simulink model "system_integration"  (R2021a)
settings: Solver=VariableStepAuto  StartTime=0.0  StopTime=3600*5  RelTol=1e-3
undefined symbols (not defined in the file): Ion, Lithium
libraries: spsSeriesRLCBranchLib x10, spsMosfetLib x7, spsBatteryLib x6, spsVoltageMeasurementLib x6, spsBreakerLib x3, spsCurrentMeasurementLib x3, spspowerguiLib x2, spsDCMachineLib x1, spsDiodeLib x1, spsPVArrayLib x1
settings Model: Creator=hp  LastModifiedBy=hp

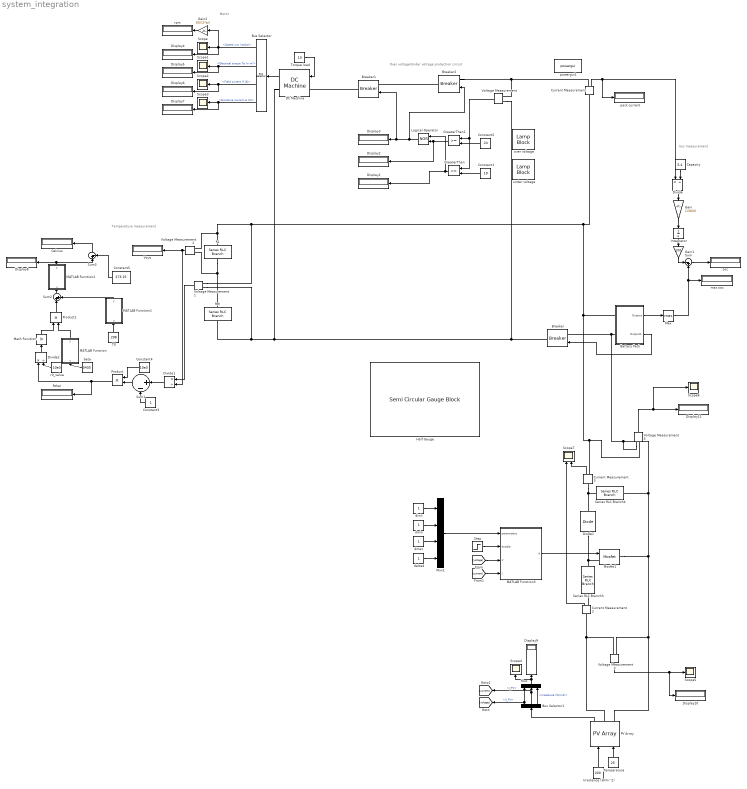
== system system_integration ==
  note: Temperature measurement
  note: Soc measurement
  note: Over voltage/Under voltage protection circuit
  note: Motor
  Battery Pack : Subsystem
  Breaker : spsBreakerLib/Breaker  InitialState=0  SwitchingTimes="[1/60  5/60]"  External=on  BreakerResistance=0.01  SnubberResistance=1e6  SnubberCapacitance=inf  Measurements=None  MoreParameters=on  NoBreakLoop=off
      settings: SourceProductBaseCode=PS
  Breaker1 : spsBreakerLib/Breaker  InitialState=0  SwitchingTimes="[1/60  5/60]"  External=on  BreakerResistance=0.01  SnubberResistance=1e6  SnubberCapacitance=inf  Measurements=None  MoreParameters=on  NoBreakLoop=off
      settings: SourceProductBaseCode=PS
  Breaker2 : spsBreakerLib/Breaker  InitialState=0  SwitchingTimes="[1/60  5/60]"  External=on  BreakerResistance=0.01  SnubberResistance=1e6  SnubberCapacitance=inf  Measurements=None  MoreParameters=on  NoBreakLoop=off
      settings: SourceProductBaseCode=PS
  Bus Selector : BusSelector  OutputSignals=Speed wm (rad/s),Electrical torque Te (n m),Field current if (A),Armature current ia (A)
  Bus Selector1 : BusSelector  OutputSignals=V_PV,I_PV,Irradiance (W/m2)
  Capacity : Constant  Value=5.4
  Celcius : Display
  Constant1 : Constant  Value=19
  Constant2 : Constant  Value=24
  Constant3 : Constant
  Constant4 : Constant  Value=10e3
  Constant5 : Constant  Value=273.15
  Current Measurement : spsCurrentMeasurementLib/Current Measurement  PhasorSimulation=off  OutputType=Complex  PSBequivalent=0
  Current Measurement2 : spsCurrentMeasurementLib/Current Measurement  PhasorSimulation=off  OutputType=Complex  PSBequivalent=0
  Current Measurement3 : spsCurrentMeasurementLib/Current Measurement  PhasorSimulation=off  OutputType=Complex  PSBequivalent=0
  DC Machine : spsDCMachineLib/DC Machine  PresetModel=No  MechanicalLoad=Torque TL  FieldType=Permanent magnet  ShowDetailedParameters=on  MeasurementBus=off  RLa="[ 0.6  0.012]"  RLf="[ 240  120]"  Laf=1.8  MachineConstant=Torque constant (N.m/A)  Ke=1.8  Kt=1.8  J=1  Bm=0  Tf=0  w0=1  Ifinit=1  TsPowergui=0  TsBlock=-1
  Diode1 : spsDiodeLib/Diode  Ron=0.001  Lon=0  Vf=0.8  IC=0  UseSnubber=0  Rs=500  Cs=250e-9  Measurements=off
  Display{1..11} (11 alike) : Display
  Divide : Product  Inputs=*/
  Divide1 : Product  Inputs=*/
  Divide2 : Product  Inputs=*/
  Gain : Gain  Gain=1/3600
  Gain1 : Gain  Gain=100
  Gain2 : Gain  Gain=60/(2*pi)
  GreaterThan : RelationalOperator  Operator=<=  OutDataTypeStr=boolean  RndMeth=Simplest
  GreaterThan1 : RelationalOperator  OutDataTypeStr=boolean  RndMeth=Simplest
  Half Gauge : SemiCircularGaugeBlock
  Integrator : Integrator
  Irradiance (W/m^2) : Constant  Value=200
  Logical Operator : Logic  Operator=NOR  AllPortsSameDT=off  OutDataTypeStr=boolean
  MATLAB Function : MATLAB Function  TreatAsAtomicUnit=on
  MATLAB Function1 : MATLAB Function  TreatAsAtomicUnit=on
  MATLAB Function2 : MATLAB Function  TreatAsAtomicUnit=on
  MATLAB Function3 : MATLAB Function  TreatAsAtomicUnit=on
  Math Function : Math  Operator=log  SaturateOnIntegerOverflow=on
  Max : MinMax  Function=max
  Mosfet1 : spsMosfetLib/Mosfet  Ron=0.1  Lon=0  Rd=0.01  Vfd=0  IC=0  Rs=1e5  Cs=inf  Measurements=off
  Mux : Mux  Inputs=3
  Mux1 : Mux
  PV Array : spsPVArrayLib/PV Array  Npar=40  Nser=10  PlotType=array @ 1000 W/m2 & specified temperatures  S_vec="[ 1000  500  100 ]"  Temp_C_vec=[45 25]  ModuleName=A10Green Technology A10J-S72-180  PlotWhenSelected=off  Pm=179.928  Ncell=72  Voc=44.06  Isc=5.31  Vm=36.72  Im=4.9  beta_Voc_pc=-0.3616  alpha_Isc_pc=0.041507  beta_Voc=-0.15932  alpha_Isc=0.002204  IL=5.3186  I0=1.8308e-10  nI=0.99015  Rsh=227.068  Rs=0.36738  RobustModel=off  RobustCellTemperature=313.3991  BAL=on  Tc=1e-6  Tfilter=5e-5
  Product : Product
  Product1 : Product
  R1 : spsSeriesRLCBranchLib/Series RLC Branch  LConnTagsString=__new0  RConnTagsString=__new0  BranchType=R  Resistance=10e3  Inductance=1e-3  SetiL0=off  InitialCurrent=0  Capacitance=1e-6  Setx0=off  InitialVoltage=0  Measurements=None
  Rth : spsSeriesRLCBranchLib/Series RLC Branch  LConnTagsString=__new0  RConnTagsString=__new0  BranchType=R  Resistance=5625  Inductance=1e-3  SetiL0=off  InitialCurrent=0  Capacitance=1e-6  Setx0=off  InitialVoltage=0  Measurements=None
  Rther : Display
  Scope{,1..6} (7 alike) : Scope
  Scope7 : Scope  NumInputPorts=2
  Series RLC Branch3 : spsSeriesRLCBranchLib/Series RLC Branch  LConnTagsString=__new0  RConnTagsString=__new0  BranchType=L  Resistance=1  Inductance=1e-3  SetiL0=off  InitialCurrent=0  Capacitance=1e-6  Setx0=off  InitialVoltage=0  Measurements=None
  Series RLC Branch4 : spsSeriesRLCBranchLib/Series RLC Branch  LConnTagsString=__new0  RConnTagsString=__new0  BranchType=C  Resistance=1  Inductance=1e-3  SetiL0=off  InitialCurrent=0  Capacitance=100e-6  Setx0=off  InitialVoltage=0  Measurements=None
  Step : Step  Time=0.0001  SampleTime=0
  Sum : Sum  Inputs=|-+
  Sum1 : Sum  Inputs=|+-
  Sum2 : Sum  Inputs=|++
  Sum3 : Sum  Inputs=|+-
  T0 : Constant  Value=298
  Temperature : Constant  Value=25
  Torque load : Constant  Value=10
  Voltage Measurement{,1..4} (5 alike) : spsVoltageMeasurementLib/Voltage Measurement  PhasorSimulation=off  OutputType=Complex  PSBequivalent=0
  Vout : Display
  beta : Constant  Value=3435
  deltad : Constant
  dinit : Constant
  dmax : Constant
  dmin : Constant
  max soc : Display
  over voltage : LampBlock
  pack current : Display
  powergui1 : spspowerguiLib/powergui  Priority=1  SimulationMode=Discrete  SampleTime=100e-6  frequency=60  Iterations=50  frequencyindice=0  Pbase=100e6  ErrMax=1e-4  UnitsV=kV  UnitsW=MW  buscounter=0  FunctionMessages=off  echomessages=off  EnableUseOfTLC=off  CurrentSourceSwitches=off  DisableSnubberDevices=off  DisableRonSwitches=off  DisableVfSwitches=off  DisplayEquations=off  AutomaticDiscreteSolvers=off  SolverType=Tustin/Backward Euler (TBE)  Interpol=off  ExternalGateDelay=off  methode=off  Ts=100  x0status=blocks  SPID=on  SwTol=0  HookPort=off  NonlinearTolerance=1e-4  nMaxIteration=100  ContinueOnMaxIteration=off  RestoreLinks=warning  ResistiveCurrentMeasurement=off  Frange=[0:2:500]  Ylog=off  Xlog=on  ShowGrid=off  save=off  variable=ZData  structure=0  ZoomFFT=off  StartTime=0.0  cycles=1  DisplayStyle=1  fundamental=60  FreqAxis=off  MaxFrequency=1000  frequencyindicesteady=1  RmsSteady=1  display=off
  r0_value : Constant  Value=10e3
  rpm : Display
  soc : Display
  under voltage : LampBlock
  wires:
  Capacity/1 -> Divide/2
  Current Measurement/1 -> pack current/1, Divide/1
  Divide/1 -> Gain/1
  Gain/1 -> Integrator/1
  Max/1 -> Sum/2, max soc/1
  Battery Pack/1(Outport) -> Max/1
  Sum/1 -> soc/1
  Integrator/1 -> Gain1/1
  Gain1/1 -> Sum/1
  Voltage Measurement/1 -> GreaterThan1/1, GreaterThan/1
  Constant1/1 -> GreaterThan/2
  Constant2/1 -> GreaterThan1/2
  GreaterThan/1 -> Display1/1, Logical Operator/1
  GreaterThan1/1 -> Display2/1, Logical Operator/2
  Logical Operator/1 -> Breaker2/1, Breaker1/1, Display3/1
  Bus Selector/4 -> Display7/1, Scope3/1  "<Armature current ia (A)>"
  Bus Selector/3 -> Display6/1, Scope2/1  "<Field current if (A)>"
  DC Machine/1 -> Bus Selector/1
  Bus Selector/2 -> Display5/1, Scope1/1  "<Electrical torque Te (n m)>"
  Gain2/1 -> rpm/1
  Bus Selector/1 -> Gain2/1, Display4/1, Scope/1  "<Speed wm (rad/s)>"
  Divide2/1 -> Math Function/1
  MATLAB Function2/1(y) -> Sum3/1, Display8/1
  Sum3/1 -> Celcius/1
  Constant5/1 -> Sum3/2
  Sum1/1 -> Product/2
  Product/1 -> Rther/1, Divide2/1
  Voltage Measurement1/1 -> Divide1/1
  beta/1 -> MATLAB Function/1(u)
  Constant4/1 -> Product/1
  Voltage Measurement2/1 -> Vout/1, Divide1/2
  T0/1 -> MATLAB Function1/1(u)
  Constant3/1 -> Sum1/2
  MATLAB Function1/1(y) -> Sum2/2
  Sum2/1 -> MATLAB Function2/1(u)
  r0_value/1 -> Divide2/2
  Product1/1 -> Sum2/1
  Divide1/1 -> Sum1/1
  Torque load/1 -> DC Machine/1
  MATLAB Function/1(y) -> Product1/2
  Math Function/1 -> Product1/1
  Battery Pack/2(Outport1) -> Breaker/1
  Mux/1 -> Scope4/1, Display9/1
  [voltage] -> MATLAB Function3/3(V)
  Step/1 -> MATLAB Function3/2(enable)
  Voltage Measurement4/1 -> Scope6/1, Display11/1
  dinit/1 -> Mux1/1
  Bus Selector1/3 -> Mux/3  "<Irradiance (W/m2)>"
  [current] -> MATLAB Function3/4(I)
  Mux1/1 -> MATLAB Function3/1(parameters)
  Bus Selector1/1 -> Mux/1, [voltage]  "<V_PV>"
  Temperature/1 -> PV Array/2
  Voltage Measurement3/1 -> Display10/1, Scope5/1
  Current Measurement2/1 -> Scope7/1
  dmin/1 -> Mux1/2
  Current Measurement3/1 -> Scope7/2
  deltad/1 -> Mux1/4
  dmax/1 -> Mux1/3
  Irradiance (W/m^2)/1 -> PV Array/1
  PV Array/1 -> Bus Selector1/1
  Bus Selector1/2 -> Mux/2, [current]  "<I_PV>"
  MATLAB Function3/1(d) -> Mosfet1/1
  connections:
  Voltage Measurement1/LConn2 -- Breaker/RConn1 -- Voltage Measurement/LConn2 -- DC Machine/RConn1 -- Rth/RConn1
  Breaker2/LConn1 -- Current Measurement/RConn1 -- Voltage Measurement/LConn1
  Breaker1/RConn1 -- DC Machine/LConn1
  Breaker2/RConn1 -- Breaker1/LConn1
  R1/RConn1 -- Rth/LConn1 -- Voltage Measurement2/LConn2
  Current Measurement3/RConn1 -- Current Measurement/LConn1 -- Voltage Measurement1/LConn1 -- Voltage Measurement2/LConn1 -- R1/LConn1 -- Battery Pack/LConn1 -- Voltage Measurement4/LConn1
  Voltage Measurement4/LConn2 -- Mosfet1/RConn1 -- Voltage Measurement3/LConn2 -- PV Array/RConn2 -- Series RLC Branch4/RConn1 -- Battery Pack/LConn2 -- Breaker/LConn1
  Voltage Measurement3/LConn1 -- PV Array/RConn1 -- Current Measurement2/LConn1
  Mosfet1/LConn1 -- Diode1/LConn1 -- Series RLC Branch3/RConn1
  Current Measurement3/LConn1 -- Series RLC Branch4/LConn1 -- Diode1/RConn1
  Current Measurement2/RConn1 -- Series RLC Branch3/LConn1

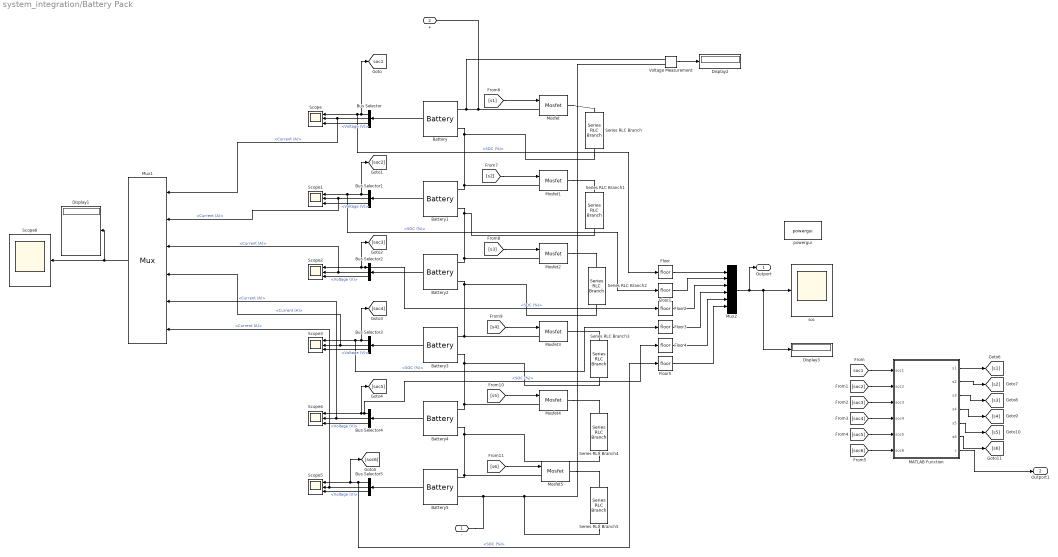
== system system_integration/Battery Pack ==
  Battery : spsBatteryLib/Battery  BatType=Lithium-Ion  ShowTempParam=off  ThermalPreset=no  ShowAgeParam=off  NomV=3.7  NomQ=5.4  SOC=65  Batt_Tr=30  PresetModel=on  MaxQ=5.4  MinV=2.775  FullV=4.3068  Dis_rate=2.3478  R=0.0068519  Normal_OP=4.8835  expZone="[3.9974      0.2653]"  current=[6.5 13 32.5]  Units=Time  Tci=20  NomT=20  T2=-30  MaxQ2=4.8  FullV2=7.1  Normal_OP2=5.655  expZone2="[6.58           1]"  Rca=0.6  ti=2000  Dp=0  Neq0=0  Tsim=1e6  Ta1=25  Qeol=5.4*0.9  Reol=0.013333*1.2  Char_age=[2.3478, 3]  Dis_age=[2.3478, 10]  N1=1500  N2=10500  N3=1000  N4=1400  Ta2=45  N5=950
  Battery1 : spsBatteryLib/Battery  BatType=Lithium-Ion  ShowTempParam=off  ThermalPreset=no  ShowAgeParam=off  NomV=3.7  NomQ=5.4  SOC=63  Batt_Tr=30  PresetModel=on  MaxQ=5.4  MinV=2.775  FullV=4.3068  Dis_rate=2.3478  R=0.0068519  Normal_OP=4.8835  expZone="[3.9974      0.2653]"  current=[6.5 13 32.5]  Units=Time  Tci=20  NomT=20  T2=-30  MaxQ2=4.8  FullV2=7.1  Normal_OP2=5.655  expZone2="[6.58           1]"  Rca=0.6  ti=2000  Dp=0  Neq0=0  Tsim=1e6  Ta1=25  Qeol=5.4*0.9  Reol=0.013333*1.2  Char_age=[2.3478, 3]  Dis_age=[2.3478, 10]  N1=1500  N2=10500  N3=1000  N4=1400  Ta2=45  N5=950
  Battery2 : spsBatteryLib/Battery  BatType=Lithium-Ion  ShowTempParam=off  ThermalPreset=no  ShowAgeParam=off  NomV=3.7  NomQ=5.4  SOC=64  Batt_Tr=30  PresetModel=on  MaxQ=5.4  MinV=2.775  FullV=4.3068  Dis_rate=2.3478  R=0.0068519  Normal_OP=4.8835  expZone="[3.9974      0.2653]"  current=[6.5 13 32.5]  Units=Time  Tci=20  NomT=20  T2=-30  MaxQ2=4.8  FullV2=7.1  Normal_OP2=5.655  expZone2="[6.58           1]"  Rca=0.6  ti=2000  Dp=0  Neq0=0  Tsim=1e6  Ta1=25  Qeol=5.4*0.9  Reol=0.013333*1.2  Char_age=[2.3478, 3]  Dis_age=[2.3478, 10]  N1=1500  N2=10500  N3=1000  N4=1400  Ta2=45  N5=950
  Battery3 : spsBatteryLib/Battery  BatType=Lithium-Ion  ShowTempParam=off  ThermalPreset=no  ShowAgeParam=off  NomV=3.7  NomQ=5.4  SOC=62  Batt_Tr=30  PresetModel=on  MaxQ=5.4  MinV=2.775  FullV=4.3068  Dis_rate=2.3478  R=0.0068519  Normal_OP=4.8835  expZone="[3.9974      0.2653]"  current=[6.5 13 32.5]  Units=Time  Tci=20  NomT=20  T2=-30  MaxQ2=4.8  FullV2=7.1  Normal_OP2=5.655  expZone2="[6.58           1]"  Rca=0.6  ti=2000  Dp=0  Neq0=0  Tsim=1e6  Ta1=25  Qeol=5.4*0.9  Reol=0.013333*1.2  Char_age=[2.3478, 3]  Dis_age=[2.3478, 10]  N1=1500  N2=10500  N3=1000  N4=1400  Ta2=45  N5=950
  Battery4 : spsBatteryLib/Battery  BatType=Lithium-Ion  ShowTempParam=off  ThermalPreset=no  ShowAgeParam=off  NomV=3.7  NomQ=5.4  SOC=66  Batt_Tr=30  PresetModel=on  MaxQ=5.4  MinV=2.775  FullV=4.3068  Dis_rate=2.3478  R=0.0068519  Normal_OP=4.8835  expZone="[3.9974      0.2653]"  current=[6.5 13 32.5]  Units=Time  Tci=20  NomT=20  T2=-30  MaxQ2=4.8  FullV2=7.1  Normal_OP2=5.655  expZone2="[6.58           1]"  Rca=0.6  ti=2000  Dp=0  Neq0=0  Tsim=1e6  Ta1=25  Qeol=5.4*0.9  Reol=0.013333*1.2  Char_age=[2.3478, 3]  Dis_age=[2.3478, 10]  N1=1500  N2=10500  N3=1000  N4=1400  Ta2=45  N5=950
  Battery5 : spsBatteryLib/Battery  BatType=Lithium-Ion  ShowTempParam=off  ThermalPreset=no  ShowAgeParam=off  NomV=3.7  NomQ=5.4  SOC=65  Batt_Tr=30  PresetModel=on  MaxQ=5.4  MinV=2.775  FullV=4.3068  Dis_rate=2.3478  R=0.0068519  Normal_OP=4.8835  expZone="[3.9974      0.2653]"  current=[6.5 13 32.5]  Units=Time  Tci=20  NomT=20  T2=-30  MaxQ2=4.8  FullV2=7.1  Normal_OP2=5.655  expZone2="[6.58           1]"  Rca=0.6  ti=2000  Dp=0  Neq0=0  Tsim=1e6  Ta1=25  Qeol=5.4*0.9  Reol=0.013333*1.2  Char_age=[2.3478, 3]  Dis_age=[2.3478, 10]  N1=1500  N2=10500  N3=1000  N4=1400  Ta2=45  N5=950
  Bus Selector{,1..5} (6 alike) : BusSelector  OutputSignals=SOC (%),Current (A),Voltage (V)
  Display1 : Display
  Display2 : Display
  Display3 : Display
  Floor{,1..5} (6 alike) : Rounding
  MATLAB Function : MATLAB Function  TreatAsAtomicUnit=on
  Mosfet{,1..5} (6 alike) : spsMosfetLib/Mosfet  Ron=0.1  Lon=0  Rd=0.01  Vfd=0  IC=0  Rs=1e5  Cs=inf  Measurements=off
  Mux1 : Mux  Inputs=6
  Mux2 : Mux  Inputs=6
  Scope{,1..5} (6 alike) : Scope  NumInputPorts=3
  Scope6 : Scope
  Series RLC Branch{,1..5} (6 alike) : spsSeriesRLCBranchLib/Series RLC Branch  LConnTagsString=__new0  RConnTagsString=__new0  BranchType=R  Resistance=0.65  Inductance=1e-3  SetiL0=off  InitialCurrent=0  Capacitance=1e-6  Setx0=off  InitialVoltage=0  Measurements=None
  Voltage Measurement : spsVoltageMeasurementLib/Voltage Measurement  PhasorSimulation=off  OutputType=Complex  PSBequivalent=0
  powergui : spspowerguiLib/powergui  Priority=1  SimulationMode=Continuous  SampleTime=0.0001  frequency=60  Iterations=50  frequencyindice=0  Pbase=100e6  ErrMax=1e-4  UnitsV=kV  UnitsW=MW  buscounter=0  FunctionMessages=off  echomessages=off  EnableUseOfTLC=off  CurrentSourceSwitches=off  DisableSnubberDevices=off  DisableRonSwitches=off  DisableVfSwitches=off  DisplayEquations=off  AutomaticDiscreteSolvers=off  SolverType=Tustin/Backward Euler (TBE)  Interpol=off  ExternalGateDelay=off  methode=off  Ts=100  x0status=blocks  SPID=on  SwTol=0  HookPort=off  NonlinearTolerance=1e-4  nMaxIteration=100  ContinueOnMaxIteration=off  RestoreLinks=warning  ResistiveCurrentMeasurement=off  Frange=[0:2:500]  Ylog=off  Xlog=on  ShowGrid=off  save=off  variable=ZData  structure=0  ZoomFFT=off  StartTime=0.0  cycles=1  DisplayStyle=1  fundamental=60  FreqAxis=off  MaxFrequency=1000  frequencyindicesteady=1  RmsSteady=1  display=off
  soc : Scope
  - : PMIOPort  Side=Left
  + : PMIOPort  Port=2  Side=Left
  Outport : Outport
  Outport1 : Outport  Port=2
  tag scope: soc1=global
  wires:
  Bus Selector5/2 -> Mux1/6, Scope5/2  "<Current (A)>"
  [s1] -> Mosfet/1
  Bus Selector5/3 -> Scope5/3  "<Voltage (V)>"
  Bus Selector2/3 -> Scope2/3  "<Voltage (V)>"
  MATLAB Function/2(s2) -> [s2]
  Bus Selector1/1 -> Floor1/1, Scope1/1, [soc2]  "<SOC (%)>"
  [soc3] -> MATLAB Function/3(soc3)
  Battery3/1 -> Bus Selector3/1
  [soc4] -> MATLAB Function/4(soc4)
  Bus Selector2/1 -> [soc3], Scope2/1, Floor2/1  "<SOC (%)>"
  Battery4/1 -> Bus Selector4/1
  Bus Selector4/1 -> Floor4/1, [soc5], Scope4/1  "<SOC (%)>"
  Battery1/1 -> Bus Selector1/1
  Bus Selector1/3 -> Scope1/3  "<Voltage (V)>"
  Bus Selector/1 -> Floor/1, Scope/1, [soc1]  "<SOC (%)>"
  Bus Selector4/2 -> Mux1/5, Scope4/2  "<Current (A)>"
  Bus Selector3/1 -> Floor3/1, Scope3/1, [soc4]  "<SOC (%)>"
  Bus Selector/2 -> Mux1/1, Scope/2  "<Current (A)>"
  Battery5/1 -> Bus Selector5/1
  [soc1] -> MATLAB Function/1(soc1)
  Bus Selector2/2 -> Mux1/3, Scope2/2  "<Current (A)>"
  Bus Selector5/1 -> Floor5/1, [soc6], Scope5/1  "<SOC (%)>"
  Battery/1 -> Bus Selector/1
  Battery2/1 -> Bus Selector2/1
  [soc2] -> MATLAB Function/2(soc2)
  Bus Selector1/2 -> Mux1/2, Scope1/2  "<Current (A)>"
  [s6] -> Mosfet5/1
  MATLAB Function/5(s5) -> [s5]
  [s4] -> Mosfet3/1
  [soc5] -> MATLAB Function/5(soc5)
  MATLAB Function/3(s3) -> [s3]
  [s5] -> Mosfet4/1
  Bus Selector3/3 -> Scope3/3  "<Voltage (V)>"
  Bus Selector/3 -> Scope/3  "<Voltage (V)>"
  [soc6] -> MATLAB Function/6(soc6)
  MATLAB Function/4(s4) -> [s4]
  Bus Selector3/2 -> Mux1/4, Scope3/2  "<Current (A)>"
  Bus Selector4/3 -> Scope4/3  "<Voltage (V)>"
  MATLAB Function/6(s6) -> [s6]
  [s3] -> Mosfet2/1
  [s2] -> Mosfet1/1
  MATLAB Function/1(s1) -> [s1]
  Mux1/1 -> Scope6/1, Display1/1
  Voltage Measurement/1 -> Display2/1
  MATLAB Function/7(c) -> Outport1/1
  Floor/1 -> Mux2/1
  Floor1/1 -> Mux2/2
  Floor2/1 -> Mux2/3
  Floor3/1 -> Mux2/4
  Floor4/1 -> Mux2/5
  Floor5/1 -> Mux2/6
  Mux2/1 -> soc/1, Display3/1, Outport/1
  connections:
  Series RLC Branch5/RConn1 -- Battery5/LConn2 -- -/RConn1 -- Voltage Measurement/LConn2
  Battery2/LConn2 -- Mosfet3/LConn1 -- Battery3/LConn1 -- Series RLC Branch2/RConn1
  Battery1/LConn2 -- Series RLC Branch1/RConn1 -- Battery2/LConn1 -- Mosfet2/LConn1
  Battery4/LConn2 -- Series RLC Branch4/RConn1 -- Mosfet5/LConn1 -- Battery5/LConn1
  Mosfet/LConn1 -- +/RConn1 -- Voltage Measurement/LConn1 -- Battery/LConn1
  Battery3/LConn2 -- Series RLC Branch3/RConn1 -- Battery4/LConn1 -- Mosfet4/LConn1
  Battery/LConn2 -- Series RLC Branch/RConn1 -- Battery1/LConn1 -- Mosfet1/LConn1
  Mosfet5/RConn1 -- Series RLC Branch5/LConn1
  Mosfet1/RConn1 -- Series RLC Branch1/LConn1
  Mosfet2/RConn1 -- Series RLC Branch2/LConn1
  Mosfet4/RConn1 -- Series RLC Branch4/LConn1
  Mosfet/RConn1 -- Series RLC Branch/LConn1
  Series RLC Branch3/LConn1 -- Mosfet3/RConn1

== matlab function system_integration/MATLAB Function ==
  data: u input; y output
function y = fcn(u)

y = (1/u);

== matlab function system_integration/Battery Pack/MATLAB Function ==
  data: soc1 input; s1 output; s2 output; soc2 input; soc3 input; soc4 input; s3 output; s4 output; soc5 input; soc6 input; s5 output; s6 output; c output
function [s1,s2,s3,s4,s5,s6,c] = fcn(soc1, soc2, soc3, soc4, soc5, soc6)
soc1=int32(soc1);
soc2=int32(soc2);
soc3=int32(soc3);
soc4=int32(soc4);
soc5=int32(soc5);
soc6=int32(soc6);
if((soc1>soc2)||(soc1>soc3)||(soc1>soc4)||(soc1>soc5)||(soc1>soc6))
    s1=1;
else
    s1=0;
end
if((soc2>soc1)||(soc2>soc3)||(soc2>soc4)||(soc2>soc5)||(soc2>soc6))
    s2=1;
else
    s2=0;
end
if((soc3>soc1)||(soc3>soc2)||(soc3>soc4)||(soc3>soc5)||(soc3>soc6))
    s3=1;
else
    s3=0;
end
if((soc4>soc1)||(soc4>soc2)||(soc4>soc3)||(soc4>soc5)||(soc4>soc6))
    s4=1;
else
    s4=0;
end
if((soc5>soc1)||(soc5>soc2)||(soc5>soc3)||(soc5>soc4)||(soc5>soc6))
    s5=1;
else
    s5=0;
end
if((soc6>soc1)||(soc6>soc2)||(soc6>soc3)||(soc6>soc4)||(soc6>soc5))
    s6=1;
else
    s6=0;
end
if((soc1==soc2)&&(soc1==soc3)&&(soc1==soc4)&&(soc1==soc5))
    s1=0; s2=0; s3=0; s4=0; s5=0; s6=0;
    c=1;
else c=0;
    
end

== matlab function system_integration/MATLAB Function1 ==
  data: u input; y output
function y = fcn(u)

y = (1/u);

== matlab function system_integration/MATLAB Function2 ==
  data: u input; y output
function y = fcn(u)

y = (1/u);

== matlab function system_integration/MATLAB Function3 ==
  data: parameters input; d output; enable input; V input; I input
function d = pando(parameters, enable, V, I)
    % Extract parameter values
    Dinit = parameters(1);
    Dmin  = parameters(2);
    Dmax  = parameters(3);
    deltad = parameters(4);

    % Declare persistent variables
    persistent vold dold pold
    if isempty(vold)
        vold = 0;
        dold = Dinit;
        pold = 0;
    end

    % Compute power
    P = V * I;

    % Control logic
    if (P - pold ~= 0 && enable ~= 0)
        if (P - pold > 0)
            if (V - vold > 0)
                d = dold - deltad;
            else
                d = dold + deltad;
            end
        elseif (P - pold < 0)
            if (V - vold < 0)
                d = dold - deltad;
            else
                d = dold + deltad;
            end
        else
            d = dold;  % Handle case where P - pold == 0
        end
    else
        d = dold;
    end

    % Clamp d within Dmin and Dmax
    d = max(min(d, Dmax), Dmin);

    % Update persistent variables
    dold = d;
    vold = V;
    pold = P;
end
